simulink model "NoC_4x4x3"  (R2015a)
settings: Solver=ode45  StartTime=0.0  StopTime=10.0  RelTol=1e-3
undefined symbols (not defined in the file or in its folder): des, SELECT
undefined symbols (not defined in the file): MAX, MIN, T
libraries: simulink x48
(part 9 of 12)

== system NoC_4x4x3/LayerUp/Sitch3DXYZ8 ==
  FIFO Queue{,1..6} (7 alike) : FIFOQueue
  Output Switch1 : OutputSwitch  NumberOutputPorts=7  SwitchingCriterion=From attribute  AttributeName=RT  InitialConditionsOpt=on  InitialConditions=5
  Path Combiner : PathCombiner  NumberInputPorts=7  InputPortPrecedence=Equiprobable  InitialSeed=13103
  RouteXYZ : Subsystem
  Single Server1 : SingleServer  ServiceTime=D  StatNumberDeparted=on
  Out_N : PMIOPort  Port=1  Side=Right
  In_N : PMIOPort  Port=2  Side=Left
  In_S : PMIOPort  Port=3  Side=Left
  Out_S : PMIOPort  Port=4  Side=Right
  In_W : PMIOPort  Port=5  Side=Left
  Out_W : PMIOPort  Port=6  Side=Right
  In_E : PMIOPort  Port=7  Side=Left
  Out_E : PMIOPort  Port=8  Side=Right
  In_U : PMIOPort  Port=9  Side=Left
  Out_U : PMIOPort  Port=10  Side=Right
  In_D : PMIOPort  Port=11  Side=Left
  In_NI : PMIOPort  Port=12  Side=Left
  Out_D : PMIOPort  Port=13  Side=Right
  Out_NI : PMIOPort  Port=14  Side=Right
  connections:
  Single Server1/LConn1 -- RouteXYZ/RConn1
  Path Combiner/RConn1 -- RouteXYZ/LConn1
  FIFO Queue6/LConn1 -- In_NI/RConn1
  FIFO Queue5/LConn1 -- In_D/RConn1
  Output Switch1/RConn7 -- Out_NI/RConn1
  Output Switch1/RConn6 -- Out_D/RConn1
  Path Combiner/LConn7 -- FIFO Queue6/RConn1
  Path Combiner/LConn6 -- FIFO Queue5/RConn1
  Out_U/RConn1 -- Output Switch1/RConn5
  Out_E/RConn1 -- Output Switch1/RConn4
  Out_W/RConn1 -- Output Switch1/RConn3
  Out_S/RConn1 -- Output Switch1/RConn2
  Out_N/RConn1 -- Output Switch1/RConn1
  Path Combiner/LConn5 -- FIFO Queue4/RConn1
  Path Combiner/LConn4 -- FIFO Queue3/RConn1
  Path Combiner/LConn3 -- FIFO Queue2/RConn1
  Path Combiner/LConn2 -- FIFO Queue1/RConn1
  Path Combiner/LConn1 -- FIFO Queue/RConn1
  Output Switch1/LConn1 -- Single Server1/RConn1
  FIFO Queue4/LConn1 -- In_U/RConn1
  FIFO Queue/LConn1 -- In_N/RConn1
  FIFO Queue3/LConn1 -- In_E/RConn1
  FIFO Queue2/LConn1 -- In_W/RConn1
  FIFO Queue1/LConn1 -- In_S/RConn1

== system NoC_4x4x3/LayerUp/Sitch3DXYZ9 ==
  FIFO Queue{,1..6} (7 alike) : FIFOQueue
  Output Switch1 : OutputSwitch  NumberOutputPorts=7  SwitchingCriterion=From attribute  AttributeName=RT  InitialConditionsOpt=on  InitialConditions=5
  Path Combiner : PathCombiner  NumberInputPorts=7  InputPortPrecedence=Equiprobable  InitialSeed=6669
  RouteXYZ : Subsystem
  Single Server1 : SingleServer  ServiceTime=D  StatNumberDeparted=on
  Out_N : PMIOPort  Port=1  Side=Right
  In_N : PMIOPort  Port=2  Side=Left
  In_S : PMIOPort  Port=3  Side=Left
  Out_S : PMIOPort  Port=4  Side=Right
  In_W : PMIOPort  Port=5  Side=Left
  Out_W : PMIOPort  Port=6  Side=Right
  In_E : PMIOPort  Port=7  Side=Left
  Out_E : PMIOPort  Port=8  Side=Right
  In_U : PMIOPort  Port=9  Side=Left
  Out_U : PMIOPort  Port=10  Side=Right
  In_D : PMIOPort  Port=11  Side=Left
  In_NI : PMIOPort  Port=12  Side=Left
  Out_D : PMIOPort  Port=13  Side=Right
  Out_NI : PMIOPort  Port=14  Side=Right
  connections:
  FIFO Queue1/LConn1 -- In_S/RConn1
  FIFO Queue2/LConn1 -- In_W/RConn1
  FIFO Queue3/LConn1 -- In_E/RConn1
  FIFO Queue/LConn1 -- In_N/RConn1
  FIFO Queue4/LConn1 -- In_U/RConn1
  Output Switch1/LConn1 -- Single Server1/RConn1
  Path Combiner/LConn1 -- FIFO Queue/RConn1
  Path Combiner/LConn2 -- FIFO Queue1/RConn1
  Path Combiner/LConn3 -- FIFO Queue2/RConn1
  Path Combiner/LConn4 -- FIFO Queue3/RConn1
  Path Combiner/LConn5 -- FIFO Queue4/RConn1
  Out_N/RConn1 -- Output Switch1/RConn1
  Out_S/RConn1 -- Output Switch1/RConn2
  Out_W/RConn1 -- Output Switch1/RConn3
  Out_E/RConn1 -- Output Switch1/RConn4
  Out_U/RConn1 -- Output Switch1/RConn5
  Path Combiner/LConn6 -- FIFO Queue5/RConn1
  Path Combiner/LConn7 -- FIFO Queue6/RConn1
  Output Switch1/RConn6 -- Out_D/RConn1
  Output Switch1/RConn7 -- Out_NI/RConn1
  FIFO Queue5/LConn1 -- In_D/RConn1
  FIFO Queue6/LConn1 -- In_NI/RConn1
  Path Combiner/RConn1 -- RouteXYZ/LConn1
  Single Server1/LConn1 -- RouteXYZ/RConn1

== system NoC_4x4x3/Layer/PE00/Create Generator Selection Variable ==
  function : TriggerPort  TriggerType=function-call
  Repeating Sequence Stair : simulink/Sources/Repeating Sequence Stair  OutValues=[0 1].'  tsamp=-1  OutMin=[]  OutMax=[]  OutDataTypeStr=float('double')  OutputDataTypeScalingMode=Specify via dialog  OutDataType=float('double')  ConRadixGroup=Best Precision: Vector-wise  OutScaling=2^-12
  Out1 : Outport
  wires:
  Repeating Sequence Stair/1 -> Out1/1

== system NoC_4x4x3/Layer/PE01/Create Generator Selection Variable ==
  function : TriggerPort  TriggerType=function-call
  Repeating Sequence Stair : simulink/Sources/Repeating Sequence Stair  OutValues=[0 1].'  tsamp=-1  OutMin=[]  OutMax=[]  OutDataTypeStr=float('double')  OutputDataTypeScalingMode=Specify via dialog  OutDataType=float('double')  ConRadixGroup=Best Precision: Vector-wise  OutScaling=2^-12
  Out1 : Outport
  wires:
  Repeating Sequence Stair/1 -> Out1/1

== system NoC_4x4x3/Layer/PE02/Create Generator Selection Variable ==
  function : TriggerPort  TriggerType=function-call
  Repeating Sequence Stair : simulink/Sources/Repeating Sequence Stair  OutValues=[0 1].'  tsamp=-1  OutMin=[]  OutMax=[]  OutDataTypeStr=float('double')  OutputDataTypeScalingMode=Specify via dialog  OutDataType=float('double')  ConRadixGroup=Best Precision: Vector-wise  OutScaling=2^-12
  Out1 : Outport
  wires:
  Repeating Sequence Stair/1 -> Out1/1

== system NoC_4x4x3/Layer/PE03/Create Generator Selection Variable ==
  function : TriggerPort  TriggerType=function-call
  Repeating Sequence Stair : simulink/Sources/Repeating Sequence Stair  OutValues=[0 1].'  tsamp=-1  OutMin=[]  OutMax=[]  OutDataTypeStr=float('double')  OutputDataTypeScalingMode=Specify via dialog  OutDataType=float('double')  ConRadixGroup=Best Precision: Vector-wise  OutScaling=2^-12
  Out1 : Outport
  wires:
  Repeating Sequence Stair/1 -> Out1/1

== system NoC_4x4x3/Layer/PE10/Create Generator Selection Variable ==
  function : TriggerPort  TriggerType=function-call
  Repeating Sequence Stair : simulink/Sources/Repeating Sequence Stair  OutValues=[0 1].'  tsamp=-1  OutMin=[]  OutMax=[]  OutDataTypeStr=float('double')  OutputDataTypeScalingMode=Specify via dialog  OutDataType=float('double')  ConRadixGroup=Best Precision: Vector-wise  OutScaling=2^-12
  Out1 : Outport
  wires:
  Repeating Sequence Stair/1 -> Out1/1

== system NoC_4x4x3/Layer/PE11/Create Generator Selection Variable ==
  function : TriggerPort  TriggerType=function-call
  Repeating Sequence Stair : simulink/Sources/Repeating Sequence Stair  OutValues=[0 1].'  tsamp=-1  OutMin=[]  OutMax=[]  OutDataTypeStr=float('double')  OutputDataTypeScalingMode=Specify via dialog  OutDataType=float('double')  ConRadixGroup=Best Precision: Vector-wise  OutScaling=2^-12
  Out1 : Outport
  wires:
  Repeating Sequence Stair/1 -> Out1/1

== system NoC_4x4x3/Layer/PE12/Create Generator Selection Variable ==
  function : TriggerPort  TriggerType=function-call
  Repeating Sequence Stair : simulink/Sources/Repeating Sequence Stair  OutValues=[0 1].'  tsamp=-1  OutMin=[]  OutMax=[]  OutDataTypeStr=float('double')  OutputDataTypeScalingMode=Specify via dialog  OutDataType=float('double')  ConRadixGroup=Best Precision: Vector-wise  OutScaling=2^-12
  Out1 : Outport
  wires:
  Repeating Sequence Stair/1 -> Out1/1

== system NoC_4x4x3/Layer/PE13/Create Generator Selection Variable ==
  function : TriggerPort  TriggerType=function-call
  Repeating Sequence Stair : simulink/Sources/Repeating Sequence Stair  OutValues=[0 1].'  tsamp=-1  OutMin=[]  OutMax=[]  OutDataTypeStr=float('double')  OutputDataTypeScalingMode=Specify via dialog  OutDataType=float('double')  ConRadixGroup=Best Precision: Vector-wise  OutScaling=2^-12
  Out1 : Outport
  wires:
  Repeating Sequence Stair/1 -> Out1/1

== system NoC_4x4x3/Layer/PE20/Create Generator Selection Variable ==
  function : TriggerPort  TriggerType=function-call
  Repeating Sequence Stair : simulink/Sources/Repeating Sequence Stair  OutValues=[0 1].'  tsamp=-1  OutMin=[]  OutMax=[]  OutDataTypeStr=float('double')  OutputDataTypeScalingMode=Specify via dialog  OutDataType=float('double')  ConRadixGroup=Best Precision: Vector-wise  OutScaling=2^-12
  Out1 : Outport
  wires:
  Repeating Sequence Stair/1 -> Out1/1

== system NoC_4x4x3/Layer/PE21/Create Generator Selection Variable ==
  function : TriggerPort  TriggerType=function-call
  Repeating Sequence Stair : simulink/Sources/Repeating Sequence Stair  OutValues=[0 1].'  tsamp=-1  OutMin=[]  OutMax=[]  OutDataTypeStr=float('double')  OutputDataTypeScalingMode=Specify via dialog  OutDataType=float('double')  ConRadixGroup=Best Precision: Vector-wise  OutScaling=2^-12
  Out1 : Outport
  wires:
  Repeating Sequence Stair/1 -> Out1/1

== system NoC_4x4x3/Layer/PE22/Create Generator Selection Variable ==
  function : TriggerPort  TriggerType=function-call
  Repeating Sequence Stair : simulink/Sources/Repeating Sequence Stair  OutValues=[0 1].'  tsamp=-1  OutMin=[]  OutMax=[]  OutDataTypeStr=float('double')  OutputDataTypeScalingMode=Specify via dialog  OutDataType=float('double')  ConRadixGroup=Best Precision: Vector-wise  OutScaling=2^-12
  Out1 : Outport
  wires:
  Repeating Sequence Stair/1 -> Out1/1

== system NoC_4x4x3/Layer/PE23/Create Generator Selection Variable ==
  function : TriggerPort  TriggerType=function-call
  Repeating Sequence Stair : simulink/Sources/Repeating Sequence Stair  OutValues=[0 1].'  tsamp=-1  OutMin=[]  OutMax=[]  OutDataTypeStr=float('double')  OutputDataTypeScalingMode=Specify via dialog  OutDataType=float('double')  ConRadixGroup=Best Precision: Vector-wise  OutScaling=2^-12
  Out1 : Outport
  wires:
  Repeating Sequence Stair/1 -> Out1/1

== system NoC_4x4x3/Layer/PE30/Create Generator Selection Variable ==
  function : TriggerPort  TriggerType=function-call
  Repeating Sequence Stair : simulink/Sources/Repeating Sequence Stair  OutValues=[0 1].'  tsamp=-1  OutMin=[]  OutMax=[]  OutDataTypeStr=float('double')  OutputDataTypeScalingMode=Specify via dialog  OutDataType=float('double')  ConRadixGroup=Best Precision: Vector-wise  OutScaling=2^-12
  Out1 : Outport
  wires:
  Repeating Sequence Stair/1 -> Out1/1

== system NoC_4x4x3/Layer/PE31/Create Generator Selection Variable ==
  function : TriggerPort  TriggerType=function-call
  Repeating Sequence Stair : simulink/Sources/Repeating Sequence Stair  OutValues=[0 1].'  tsamp=-1  OutMin=[]  OutMax=[]  OutDataTypeStr=float('double')  OutputDataTypeScalingMode=Specify via dialog  OutDataType=float('double')  ConRadixGroup=Best Precision: Vector-wise  OutScaling=2^-12
  Out1 : Outport
  wires:
  Repeating Sequence Stair/1 -> Out1/1

== system NoC_4x4x3/Layer/PE32/Create Generator Selection Variable ==
  function : TriggerPort  TriggerType=function-call
  Repeating Sequence Stair : simulink/Sources/Repeating Sequence Stair  OutValues=[0 1].'  tsamp=-1  OutMin=[]  OutMax=[]  OutDataTypeStr=float('double')  OutputDataTypeScalingMode=Specify via dialog  OutDataType=float('double')  ConRadixGroup=Best Precision: Vector-wise  OutScaling=2^-12
  Out1 : Outport
  wires:
  Repeating Sequence Stair/1 -> Out1/1

== system NoC_4x4x3/Layer/PE33/Create Generator Selection Variable ==
  function : TriggerPort  TriggerType=function-call
  Repeating Sequence Stair : simulink/Sources/Repeating Sequence Stair  OutValues=[0 1].'  tsamp=-1  OutMin=[]  OutMax=[]  OutDataTypeStr=float('double')  OutputDataTypeScalingMode=Specify via dialog  OutDataType=float('double')  ConRadixGroup=Best Precision: Vector-wise  OutScaling=2^-12
  Out1 : Outport
  wires:
  Repeating Sequence Stair/1 -> Out1/1

== system NoC_4x4x3/Layer/Sitch3DXYZ/RouteXYZ ==
  Attribute Function : Subsystem  LoadFcn=des.afb.attributefunction_support(gcb,'LoadFcn');  StartFcn=des.afb.attributefunction_support(gcb,'StartFcn');  mask(Attribute Function){OutputNamePrefix=out_}
      mask prompts: OutputNamePrefix "Prefix name"
      settings: CopyFcn=des.afb.attributefunction_support(gcb,'CopyFcn');  OpenFcn=des.afb.attributefunction_support(gcb,'OpenFcn');  ErrorFcn=des.afb.error_redirect
      mask Help: slhelp(gcbh)
      mask Display: image(des_iconLoad('attribFunction.jpg'),'center');
  Set Attribute : SetAttribute  AttributeName=IME_X|IME_Y|IME_Z  AttributeFrom=Dialog|Dialog|Dialog  AttributeValue=ME_X|ME_Y|ME_Z  AttributeTreatAsVector=1|1|1  EvaluatedAttributeValue={ ME_X;ME_Y;ME_Z}
  Input : PMIOPort  Port=1  Side=Left
  Output : PMIOPort  Port=2  Side=Right
  connections:
  Set Attribute/RConn1 -- Attribute Function/LConn1
  Output/RConn1 -- Attribute Function/RConn1
  Input/RConn1 -- Set Attribute/LConn1

== system NoC_4x4x3/Layer/Sitch3DXYZ1/RouteXYZ ==
  Attribute Function : Subsystem  LoadFcn=des.afb.attributefunction_support(gcb,'LoadFcn');  StartFcn=des.afb.attributefunction_support(gcb,'StartFcn');  mask(Attribute Function){OutputNamePrefix=out_}
      mask prompts: OutputNamePrefix "Prefix name"
      settings: CopyFcn=des.afb.attributefunction_support(gcb,'CopyFcn');  OpenFcn=des.afb.attributefunction_support(gcb,'OpenFcn');  ErrorFcn=des.afb.error_redirect
      mask Help: slhelp(gcbh)
      mask Display: image(des_iconLoad('attribFunction.jpg'),'center');
  Set Attribute : SetAttribute  AttributeName=IME_X|IME_Y|IME_Z  AttributeFrom=Dialog|Dialog|Dialog  AttributeValue=ME_X|ME_Y|ME_Z  AttributeTreatAsVector=1|1|1  EvaluatedAttributeValue={ ME_X;ME_Y;ME_Z}
  Input : PMIOPort  Port=1  Side=Left
  Output : PMIOPort  Port=2  Side=Right
  connections:
  Input/RConn1 -- Set Attribute/LConn1
  Output/RConn1 -- Attribute Function/RConn1
  Set Attribute/RConn1 -- Attribute Function/LConn1

== system NoC_4x4x3/Layer/Sitch3DXYZ10/RouteXYZ ==
  Attribute Function : Subsystem  LoadFcn=des.afb.attributefunction_support(gcb,'LoadFcn');  StartFcn=des.afb.attributefunction_support(gcb,'StartFcn');  mask(Attribute Function){OutputNamePrefix=out_}
      mask prompts: OutputNamePrefix "Prefix name"
      settings: CopyFcn=des.afb.attributefunction_support(gcb,'CopyFcn');  OpenFcn=des.afb.attributefunction_support(gcb,'OpenFcn');  ErrorFcn=des.afb.error_redirect
      mask Help: slhelp(gcbh)
      mask Display: image(des_iconLoad('attribFunction.jpg'),'center');
  Set Attribute : SetAttribute  AttributeName=IME_X|IME_Y|IME_Z  AttributeFrom=Dialog|Dialog|Dialog  AttributeValue=ME_X|ME_Y|ME_Z  AttributeTreatAsVector=1|1|1  EvaluatedAttributeValue={ ME_X;ME_Y;ME_Z}
  Input : PMIOPort  Port=1  Side=Left
  Output : PMIOPort  Port=2  Side=Right
  connections:
  Set Attribute/RConn1 -- Attribute Function/LConn1
  Output/RConn1 -- Attribute Function/RConn1
  Input/RConn1 -- Set Attribute/LConn1

== system NoC_4x4x3/Layer/Sitch3DXYZ11/RouteXYZ ==
  Attribute Function : Subsystem  LoadFcn=des.afb.attributefunction_support(gcb,'LoadFcn');  StartFcn=des.afb.attributefunction_support(gcb,'StartFcn');  mask(Attribute Function){OutputNamePrefix=out_}
      mask prompts: OutputNamePrefix "Prefix name"
      settings: CopyFcn=des.afb.attributefunction_support(gcb,'CopyFcn');  OpenFcn=des.afb.attributefunction_support(gcb,'OpenFcn');  ErrorFcn=des.afb.error_redirect
      mask Help: slhelp(gcbh)
      mask Display: image(des_iconLoad('attribFunction.jpg'),'center');
  Set Attribute : SetAttribute  AttributeName=IME_X|IME_Y|IME_Z  AttributeFrom=Dialog|Dialog|Dialog  AttributeValue=ME_X|ME_Y|ME_Z  AttributeTreatAsVector=1|1|1  EvaluatedAttributeValue={ ME_X;ME_Y;ME_Z}
  Input : PMIOPort  Port=1  Side=Left
  Output : PMIOPort  Port=2  Side=Right
  connections:
  Input/RConn1 -- Set Attribute/LConn1
  Output/RConn1 -- Attribute Function/RConn1
  Set Attribute/RConn1 -- Attribute Function/LConn1

== system NoC_4x4x3/Layer/Sitch3DXYZ12/RouteXYZ ==
  Attribute Function : Subsystem  LoadFcn=des.afb.attributefunction_support(gcb,'LoadFcn');  StartFcn=des.afb.attributefunction_support(gcb,'StartFcn');  mask(Attribute Function){OutputNamePrefix=out_}
      mask prompts: OutputNamePrefix "Prefix name"
      settings: CopyFcn=des.afb.attributefunction_support(gcb,'CopyFcn');  OpenFcn=des.afb.attributefunction_support(gcb,'OpenFcn');  ErrorFcn=des.afb.error_redirect
      mask Help: slhelp(gcbh)
      mask Display: image(des_iconLoad('attribFunction.jpg'),'center');
  Set Attribute : SetAttribute  AttributeName=IME_X|IME_Y|IME_Z  AttributeFrom=Dialog|Dialog|Dialog  AttributeValue=ME_X|ME_Y|ME_Z  AttributeTreatAsVector=1|1|1  EvaluatedAttributeValue={ ME_X;ME_Y;ME_Z}
  Input : PMIOPort  Port=1  Side=Left
  Output : PMIOPort  Port=2  Side=Right
  connections:
  Input/RConn1 -- Set Attribute/LConn1
  Output/RConn1 -- Attribute Function/RConn1
  Set Attribute/RConn1 -- Attribute Function/LConn1

== system NoC_4x4x3/Layer/Sitch3DXYZ13/RouteXYZ ==
  Attribute Function : Subsystem  LoadFcn=des.afb.attributefunction_support(gcb,'LoadFcn');  StartFcn=des.afb.attributefunction_support(gcb,'StartFcn');  mask(Attribute Function){OutputNamePrefix=out_}
      mask prompts: OutputNamePrefix "Prefix name"
      settings: CopyFcn=des.afb.attributefunction_support(gcb,'CopyFcn');  OpenFcn=des.afb.attributefunction_support(gcb,'OpenFcn');  ErrorFcn=des.afb.error_redirect
      mask Help: slhelp(gcbh)
      mask Display: image(des_iconLoad('attribFunction.jpg'),'center');
  Set Attribute : SetAttribute  AttributeName=IME_X|IME_Y|IME_Z  AttributeFrom=Dialog|Dialog|Dialog  AttributeValue=ME_X|ME_Y|ME_Z  AttributeTreatAsVector=1|1|1  EvaluatedAttributeValue={ ME_X;ME_Y;ME_Z}
  Input : PMIOPort  Port=1  Side=Left
  Output : PMIOPort  Port=2  Side=Right
  connections:
  Set Attribute/RConn1 -- Attribute Function/LConn1
  Output/RConn1 -- Attribute Function/RConn1
  Input/RConn1 -- Set Attribute/LConn1

== system NoC_4x4x3/Layer/Sitch3DXYZ14/RouteXYZ ==
  Attribute Function : Subsystem  LoadFcn=des.afb.attributefunction_support(gcb,'LoadFcn');  StartFcn=des.afb.attributefunction_support(gcb,'StartFcn');  mask(Attribute Function){OutputNamePrefix=out_}
      mask prompts: OutputNamePrefix "Prefix name"
      settings: CopyFcn=des.afb.attributefunction_support(gcb,'CopyFcn');  OpenFcn=des.afb.attributefunction_support(gcb,'OpenFcn');  ErrorFcn=des.afb.error_redirect
      mask Help: slhelp(gcbh)
      mask Display: image(des_iconLoad('attribFunction.jpg'),'center');
  Set Attribute : SetAttribute  AttributeName=IME_X|IME_Y|IME_Z  AttributeFrom=Dialog|Dialog|Dialog  AttributeValue=ME_X|ME_Y|ME_Z  AttributeTreatAsVector=1|1|1  EvaluatedAttributeValue={ ME_X;ME_Y;ME_Z}
  Input : PMIOPort  Port=1  Side=Left
  Output : PMIOPort  Port=2  Side=Right
  connections:
  Input/RConn1 -- Set Attribute/LConn1
  Output/RConn1 -- Attribute Function/RConn1
  Set Attribute/RConn1 -- Attribute Function/LConn1

== system NoC_4x4x3/Layer/Sitch3DXYZ15/RouteXYZ ==
  Attribute Function : Subsystem  LoadFcn=des.afb.attributefunction_support(gcb,'LoadFcn');  StartFcn=des.afb.attributefunction_support(gcb,'StartFcn');  mask(Attribute Function){OutputNamePrefix=out_}
      mask prompts: OutputNamePrefix "Prefix name"
      settings: CopyFcn=des.afb.attributefunction_support(gcb,'CopyFcn');  OpenFcn=des.afb.attributefunction_support(gcb,'OpenFcn');  ErrorFcn=des.afb.error_redirect
      mask Help: slhelp(gcbh)
      mask Display: image(des_iconLoad('attribFunction.jpg'),'center');
  Set Attribute : SetAttribute  AttributeName=IME_X|IME_Y|IME_Z  AttributeFrom=Dialog|Dialog|Dialog  AttributeValue=ME_X|ME_Y|ME_Z  AttributeTreatAsVector=1|1|1  EvaluatedAttributeValue={ ME_X;ME_Y;ME_Z}
  Input : PMIOPort  Port=1  Side=Left
  Output : PMIOPort  Port=2  Side=Right
  connections:
  Set Attribute/RConn1 -- Attribute Function/LConn1
  Output/RConn1 -- Attribute Function/RConn1
  Input/RConn1 -- Set Attribute/LConn1

== system NoC_4x4x3/Layer/Sitch3DXYZ2/RouteXYZ ==
  Attribute Function : Subsystem  LoadFcn=des.afb.attributefunction_support(gcb,'LoadFcn');  StartFcn=des.afb.attributefunction_support(gcb,'StartFcn');  mask(Attribute Function){OutputNamePrefix=out_}
      mask prompts: OutputNamePrefix "Prefix name"
      settings: CopyFcn=des.afb.attributefunction_support(gcb,'CopyFcn');  OpenFcn=des.afb.attributefunction_support(gcb,'OpenFcn');  ErrorFcn=des.afb.error_redirect
      mask Help: slhelp(gcbh)
      mask Display: image(des_iconLoad('attribFunction.jpg'),'center');
  Set Attribute : SetAttribute  AttributeName=IME_X|IME_Y|IME_Z  AttributeFrom=Dialog|Dialog|Dialog  AttributeValue=ME_X|ME_Y|ME_Z  AttributeTreatAsVector=1|1|1  EvaluatedAttributeValue={ ME_X;ME_Y;ME_Z}
  Input : PMIOPort  Port=1  Side=Left
  Output : PMIOPort  Port=2  Side=Right
  connections:
  Set Attribute/RConn1 -- Attribute Function/LConn1
  Output/RConn1 -- Attribute Function/RConn1
  Input/RConn1 -- Set Attribute/LConn1

== system NoC_4x4x3/Layer/Sitch3DXYZ3/RouteXYZ ==
  Attribute Function : Subsystem  LoadFcn=des.afb.attributefunction_support(gcb,'LoadFcn');  StartFcn=des.afb.attributefunction_support(gcb,'StartFcn');  mask(Attribute Function){OutputNamePrefix=out_}
      mask prompts: OutputNamePrefix "Prefix name"
      settings: CopyFcn=des.afb.attributefunction_support(gcb,'CopyFcn');  OpenFcn=des.afb.attributefunction_support(gcb,'OpenFcn');  ErrorFcn=des.afb.error_redirect
      mask Help: slhelp(gcbh)
      mask Display: image(des_iconLoad('attribFunction.jpg'),'center');
  Set Attribute : SetAttribute  AttributeName=IME_X|IME_Y|IME_Z  AttributeFrom=Dialog|Dialog|Dialog  AttributeValue=ME_X|ME_Y|ME_Z  AttributeTreatAsVector=1|1|1  EvaluatedAttributeValue={ ME_X;ME_Y;ME_Z}
  Input : PMIOPort  Port=1  Side=Left
  Output : PMIOPort  Port=2  Side=Right
  connections:
  Input/RConn1 -- Set Attribute/LConn1
  Output/RConn1 -- Attribute Function/RConn1
  Set Attribute/RConn1 -- Attribute Function/LConn1

== system NoC_4x4x3/Layer/Sitch3DXYZ4/RouteXYZ ==
  Attribute Function : Subsystem  LoadFcn=des.afb.attributefunction_support(gcb,'LoadFcn');  StartFcn=des.afb.attributefunction_support(gcb,'StartFcn');  mask(Attribute Function){OutputNamePrefix=out_}
      mask prompts: OutputNamePrefix "Prefix name"
      settings: CopyFcn=des.afb.attributefunction_support(gcb,'CopyFcn');  OpenFcn=des.afb.attributefunction_support(gcb,'OpenFcn');  ErrorFcn=des.afb.error_redirect
      mask Help: slhelp(gcbh)
      mask Display: image(des_iconLoad('attribFunction.jpg'),'center');
  Set Attribute : SetAttribute  AttributeName=IME_X|IME_Y|IME_Z  AttributeFrom=Dialog|Dialog|Dialog  AttributeValue=ME_X|ME_Y|ME_Z  AttributeTreatAsVector=1|1|1  EvaluatedAttributeValue={ ME_X;ME_Y;ME_Z}
  Input : PMIOPort  Port=1  Side=Left
  Output : PMIOPort  Port=2  Side=Right
  connections:
  Input/RConn1 -- Set Attribute/LConn1
  Output/RConn1 -- Attribute Function/RConn1
  Set Attribute/RConn1 -- Attribute Function/LConn1

== system NoC_4x4x3/Layer/Sitch3DXYZ5/RouteXYZ ==
  Attribute Function : Subsystem  LoadFcn=des.afb.attributefunction_support(gcb,'LoadFcn');  StartFcn=des.afb.attributefunction_support(gcb,'StartFcn');  mask(Attribute Function){OutputNamePrefix=out_}
      mask prompts: OutputNamePrefix "Prefix name"
      settings: CopyFcn=des.afb.attributefunction_support(gcb,'CopyFcn');  OpenFcn=des.afb.attributefunction_support(gcb,'OpenFcn');  ErrorFcn=des.afb.error_redirect
      mask Help: slhelp(gcbh)
      mask Display: image(des_iconLoad('attribFunction.jpg'),'center');
  Set Attribute : SetAttribute  AttributeName=IME_X|IME_Y|IME_Z  AttributeFrom=Dialog|Dialog|Dialog  AttributeValue=ME_X|ME_Y|ME_Z  AttributeTreatAsVector=1|1|1  EvaluatedAttributeValue={ ME_X;ME_Y;ME_Z}
  Input : PMIOPort  Port=1  Side=Left
  Output : PMIOPort  Port=2  Side=Right
  connections:
  Set Attribute/RConn1 -- Attribute Function/LConn1
  Output/RConn1 -- Attribute Function/RConn1
  Input/RConn1 -- Set Attribute/LConn1

== system NoC_4x4x3/Layer/Sitch3DXYZ6/RouteXYZ ==
  Attribute Function : Subsystem  LoadFcn=des.afb.attributefunction_support(gcb,'LoadFcn');  StartFcn=des.afb.attributefunction_support(gcb,'StartFcn');  mask(Attribute Function){OutputNamePrefix=out_}
      mask prompts: OutputNamePrefix "Prefix name"
      settings: CopyFcn=des.afb.attributefunction_support(gcb,'CopyFcn');  OpenFcn=des.afb.attributefunction_support(gcb,'OpenFcn');  ErrorFcn=des.afb.error_redirect
      mask Help: slhelp(gcbh)
      mask Display: image(des_iconLoad('attribFunction.jpg'),'center');
  Set Attribute : SetAttribute  AttributeName=IME_X|IME_Y|IME_Z  AttributeFrom=Dialog|Dialog|Dialog  AttributeValue=ME_X|ME_Y|ME_Z  AttributeTreatAsVector=1|1|1  EvaluatedAttributeValue={ ME_X;ME_Y;ME_Z}
  Input : PMIOPort  Port=1  Side=Left
  Output : PMIOPort  Port=2  Side=Right
  connections:
  Input/RConn1 -- Set Attribute/LConn1
  Output/RConn1 -- Attribute Function/RConn1
  Set Attribute/RConn1 -- Attribute Function/LConn1

== system NoC_4x4x3/Layer/Sitch3DXYZ7/RouteXYZ ==
  Attribute Function : Subsystem  LoadFcn=des.afb.attributefunction_support(gcb,'LoadFcn');  StartFcn=des.afb.attributefunction_support(gcb,'StartFcn');  mask(Attribute Function){OutputNamePrefix=out_}
      mask prompts: OutputNamePrefix "Prefix name"
      settings: CopyFcn=des.afb.attributefunction_support(gcb,'CopyFcn');  OpenFcn=des.afb.attributefunction_support(gcb,'OpenFcn');  ErrorFcn=des.afb.error_redirect
      mask Help: slhelp(gcbh)
      mask Display: image(des_iconLoad('attribFunction.jpg'),'center');
  Set Attribute : SetAttribute  AttributeName=IME_X|IME_Y|IME_Z  AttributeFrom=Dialog|Dialog|Dialog  AttributeValue=ME_X|ME_Y|ME_Z  AttributeTreatAsVector=1|1|1  EvaluatedAttributeValue={ ME_X;ME_Y;ME_Z}
  Input : PMIOPort  Port=1  Side=Left
  Output : PMIOPort  Port=2  Side=Right
  connections:
  Set Attribute/RConn1 -- Attribute Function/LConn1
  Output/RConn1 -- Attribute Function/RConn1
  Input/RConn1 -- Set Attribute/LConn1

== system NoC_4x4x3/Layer/Sitch3DXYZ8/RouteXYZ ==
  Attribute Function : Subsystem  LoadFcn=des.afb.attributefunction_support(gcb,'LoadFcn');  StartFcn=des.afb.attributefunction_support(gcb,'StartFcn');  mask(Attribute Function){OutputNamePrefix=out_}
      mask prompts: OutputNamePrefix "Prefix name"
      settings: CopyFcn=des.afb.attributefunction_support(gcb,'CopyFcn');  OpenFcn=des.afb.attributefunction_support(gcb,'OpenFcn');  ErrorFcn=des.afb.error_redirect
      mask Help: slhelp(gcbh)
      mask Display: image(des_iconLoad('attribFunction.jpg'),'center');
  Set Attribute : SetAttribute  AttributeName=IME_X|IME_Y|IME_Z  AttributeFrom=Dialog|Dialog|Dialog  AttributeValue=ME_X|ME_Y|ME_Z  AttributeTreatAsVector=1|1|1  EvaluatedAttributeValue={ ME_X;ME_Y;ME_Z}
  Input : PMIOPort  Port=1  Side=Left
  Output : PMIOPort  Port=2  Side=Right
  connections:
  Set Attribute/RConn1 -- Attribute Function/LConn1
  Output/RConn1 -- Attribute Function/RConn1
  Input/RConn1 -- Set Attribute/LConn1

== system NoC_4x4x3/Layer/Sitch3DXYZ9/RouteXYZ ==
  Attribute Function : Subsystem  LoadFcn=des.afb.attributefunction_support(gcb,'LoadFcn');  StartFcn=des.afb.attributefunction_support(gcb,'StartFcn');  mask(Attribute Function){OutputNamePrefix=out_}
      mask prompts: OutputNamePrefix "Prefix name"
      settings: CopyFcn=des.afb.attributefunction_support(gcb,'CopyFcn');  OpenFcn=des.afb.attributefunction_support(gcb,'OpenFcn');  ErrorFcn=des.afb.error_redirect
      mask Help: slhelp(gcbh)
      mask Display: image(des_iconLoad('attribFunction.jpg'),'center');
  Set Attribute : SetAttribute  AttributeName=IME_X|IME_Y|IME_Z  AttributeFrom=Dialog|Dialog|Dialog  AttributeValue=ME_X|ME_Y|ME_Z  AttributeTreatAsVector=1|1|1  EvaluatedAttributeValue={ ME_X;ME_Y;ME_Z}
  Input : PMIOPort  Port=1  Side=Left
  Output : PMIOPort  Port=2  Side=Right
  connections:
  Input/RConn1 -- Set Attribute/LConn1
  Output/RConn1 -- Attribute Function/RConn1
  Set Attribute/RConn1 -- Attribute Function/LConn1

== system NoC_4x4x3/LayerDown/PE00/Create Generator Selection Variable ==
  function : TriggerPort  TriggerType=function-call
  Repeating Sequence Stair : simulink/Sources/Repeating Sequence Stair  OutValues=[0 1].'  tsamp=-1  OutMin=[]  OutMax=[]  OutDataTypeStr=float('double')  OutputDataTypeScalingMode=Specify via dialog  OutDataType=float('double')  ConRadixGroup=Best Precision: Vector-wise  OutScaling=2^-12
  Out1 : Outport
  wires:
  Repeating Sequence Stair/1 -> Out1/1

== system NoC_4x4x3/LayerDown/PE01/Create Generator Selection Variable ==
  function : TriggerPort  TriggerType=function-call
  Repeating Sequence Stair : simulink/Sources/Repeating Sequence Stair  OutValues=[0 1].'  tsamp=-1  OutMin=[]  OutMax=[]  OutDataTypeStr=float('double')  OutputDataTypeScalingMode=Specify via dialog  OutDataType=float('double')  ConRadixGroup=Best Precision: Vector-wise  OutScaling=2^-12
  Out1 : Outport
  wires:
  Repeating Sequence Stair/1 -> Out1/1

== system NoC_4x4x3/LayerDown/PE02/Create Generator Selection Variable ==
  function : TriggerPort  TriggerType=function-call
  Repeating Sequence Stair : simulink/Sources/Repeating Sequence Stair  OutValues=[0 1].'  tsamp=-1  OutMin=[]  OutMax=[]  OutDataTypeStr=float('double')  OutputDataTypeScalingMode=Specify via dialog  OutDataType=float('double')  ConRadixGroup=Best Precision: Vector-wise  OutScaling=2^-12
  Out1 : Outport
  wires:
  Repeating Sequence Stair/1 -> Out1/1

== system NoC_4x4x3/LayerDown/PE03/Create Generator Selection Variable ==
  function : TriggerPort  TriggerType=function-call
  Repeating Sequence Stair : simulink/Sources/Repeating Sequence Stair  OutValues=[0 1].'  tsamp=-1  OutMin=[]  OutMax=[]  OutDataTypeStr=float('double')  OutputDataTypeScalingMode=Specify via dialog  OutDataType=float('double')  ConRadixGroup=Best Precision: Vector-wise  OutScaling=2^-12
  Out1 : Outport
  wires:
  Repeating Sequence Stair/1 -> Out1/1

== system NoC_4x4x3/LayerDown/PE10/Create Generator Selection Variable ==
  function : TriggerPort  TriggerType=function-call
  Repeating Sequence Stair : simulink/Sources/Repeating Sequence Stair  OutValues=[0 1].'  tsamp=-1  OutMin=[]  OutMax=[]  OutDataTypeStr=float('double')  OutputDataTypeScalingMode=Specify via dialog  OutDataType=float('double')  ConRadixGroup=Best Precision: Vector-wise  OutScaling=2^-12
  Out1 : Outport
  wires:
  Repeating Sequence Stair/1 -> Out1/1

== system NoC_4x4x3/LayerDown/PE11/Create Generator Selection Variable ==
  function : TriggerPort  TriggerType=function-call
  Repeating Sequence Stair : simulink/Sources/Repeating Sequence Stair  OutValues=[0 1].'  tsamp=-1  OutMin=[]  OutMax=[]  OutDataTypeStr=float('double')  OutputDataTypeScalingMode=Specify via dialog  OutDataType=float('double')  ConRadixGroup=Best Precision: Vector-wise  OutScaling=2^-12
  Out1 : Outport
  wires:
  Repeating Sequence Stair/1 -> Out1/1

== system NoC_4x4x3/LayerDown/PE12/Create Generator Selection Variable ==
  function : TriggerPort  TriggerType=function-call
  Repeating Sequence Stair : simulink/Sources/Repeating Sequence Stair  OutValues=[0 1].'  tsamp=-1  OutMin=[]  OutMax=[]  OutDataTypeStr=float('double')  OutputDataTypeScalingMode=Specify via dialog  OutDataType=float('double')  ConRadixGroup=Best Precision: Vector-wise  OutScaling=2^-12
  Out1 : Outport
  wires:
  Repeating Sequence Stair/1 -> Out1/1

== system NoC_4x4x3/LayerDown/PE13/Create Generator Selection Variable ==
  function : TriggerPort  TriggerType=function-call
  Repeating Sequence Stair : simulink/Sources/Repeating Sequence Stair  OutValues=[0 1].'  tsamp=-1  OutMin=[]  OutMax=[]  OutDataTypeStr=float('double')  OutputDataTypeScalingMode=Specify via dialog  OutDataType=float('double')  ConRadixGroup=Best Precision: Vector-wise  OutScaling=2^-12
  Out1 : Outport
  wires:
  Repeating Sequence Stair/1 -> Out1/1

== system NoC_4x4x3/LayerDown/PE20/Create Generator Selection Variable ==
  function : TriggerPort  TriggerType=function-call
  Repeating Sequence Stair : simulink/Sources/Repeating Sequence Stair  OutValues=[0 1].'  tsamp=-1  OutMin=[]  OutMax=[]  OutDataTypeStr=float('double')  OutputDataTypeScalingMode=Specify via dialog  OutDataType=float('double')  ConRadixGroup=Best Precision: Vector-wise  OutScaling=2^-12
  Out1 : Outport
  wires:
  Repeating Sequence Stair/1 -> Out1/1

== system NoC_4x4x3/LayerDown/PE21/Create Generator Selection Variable ==
  function : TriggerPort  TriggerType=function-call
  Repeating Sequence Stair : simulink/Sources/Repeating Sequence Stair  OutValues=[0 1].'  tsamp=-1  OutMin=[]  OutMax=[]  OutDataTypeStr=float('double')  OutputDataTypeScalingMode=Specify via dialog  OutDataType=float('double')  ConRadixGroup=Best Precision: Vector-wise  OutScaling=2^-12
  Out1 : Outport
  wires:
  Repeating Sequence Stair/1 -> Out1/1

== system NoC_4x4x3/LayerDown/PE22/Create Generator Selection Variable ==
  function : TriggerPort  TriggerType=function-call
  Repeating Sequence Stair : simulink/Sources/Repeating Sequence Stair  OutValues=[0 1].'  tsamp=-1  OutMin=[]  OutMax=[]  OutDataTypeStr=float('double')  OutputDataTypeScalingMode=Specify via dialog  OutDataType=float('double')  ConRadixGroup=Best Precision: Vector-wise  OutScaling=2^-12
  Out1 : Outport
  wires:
  Repeating Sequence Stair/1 -> Out1/1

== system NoC_4x4x3/LayerDown/PE23/Create Generator Selection Variable ==
  function : TriggerPort  TriggerType=function-call
  Repeating Sequence Stair : simulink/Sources/Repeating Sequence Stair  OutValues=[0 1].'  tsamp=-1  OutMin=[]  OutMax=[]  OutDataTypeStr=float('double')  OutputDataTypeScalingMode=Specify via dialog  OutDataType=float('double')  ConRadixGroup=Best Precision: Vector-wise  OutScaling=2^-12
  Out1 : Outport
  wires:
  Repeating Sequence Stair/1 -> Out1/1

== system NoC_4x4x3/LayerDown/PE30/Create Generator Selection Variable ==
  function : TriggerPort  TriggerType=function-call
  Repeating Sequence Stair : simulink/Sources/Repeating Sequence Stair  OutValues=[0 1].'  tsamp=-1  OutMin=[]  OutMax=[]  OutDataTypeStr=float('double')  OutputDataTypeScalingMode=Specify via dialog  OutDataType=float('double')  ConRadixGroup=Best Precision: Vector-wise  OutScaling=2^-12
  Out1 : Outport
  wires:
  Repeating Sequence Stair/1 -> Out1/1

== system NoC_4x4x3/LayerDown/PE31/Create Generator Selection Variable ==
  function : TriggerPort  TriggerType=function-call
  Repeating Sequence Stair : simulink/Sources/Repeating Sequence Stair  OutValues=[0 1].'  tsamp=-1  OutMin=[]  OutMax=[]  OutDataTypeStr=float('double')  OutputDataTypeScalingMode=Specify via dialog  OutDataType=float('double')  ConRadixGroup=Best Precision: Vector-wise  OutScaling=2^-12
  Out1 : Outport
  wires:
  Repeating Sequence Stair/1 -> Out1/1

== system NoC_4x4x3/LayerDown/PE32/Create Generator Selection Variable ==
  function : TriggerPort  TriggerType=function-call
  Repeating Sequence Stair : simulink/Sources/Repeating Sequence Stair  OutValues=[0 1].'  tsamp=-1  OutMin=[]  OutMax=[]  OutDataTypeStr=float('double')  OutputDataTypeScalingMode=Specify via dialog  OutDataType=float('double')  ConRadixGroup=Best Precision: Vector-wise  OutScaling=2^-12
  Out1 : Outport
  wires:
  Repeating Sequence Stair/1 -> Out1/1

== system NoC_4x4x3/LayerDown/PE33/Create Generator Selection Variable ==
  function : TriggerPort  TriggerType=function-call
  Repeating Sequence Stair : simulink/Sources/Repeating Sequence Stair  OutValues=[0 1].'  tsamp=-1  OutMin=[]  OutMax=[]  OutDataTypeStr=float('double')  OutputDataTypeScalingMode=Specify via dialog  OutDataType=float('double')  ConRadixGroup=Best Precision: Vector-wise  OutScaling=2^-12
  Out1 : Outport
  wires:
  Repeating Sequence Stair/1 -> Out1/1

== system NoC_4x4x3/LayerDown/Sitch3DXYZ/RouteXYZ ==
  Attribute Function : Subsystem  LoadFcn=des.afb.attributefunction_support(gcb,'LoadFcn');  StartFcn=des.afb.attributefunction_support(gcb,'StartFcn');  mask(Attribute Function){OutputNamePrefix=out_}
      mask prompts: OutputNamePrefix "Prefix name"
      settings: CopyFcn=des.afb.attributefunction_support(gcb,'CopyFcn');  OpenFcn=des.afb.attributefunction_support(gcb,'OpenFcn');  ErrorFcn=des.afb.error_redirect
      mask Help: slhelp(gcbh)
      mask Display: image(des_iconLoad('attribFunction.jpg'),'center');
  Set Attribute : SetAttribute  AttributeName=IME_X|IME_Y|IME_Z  AttributeFrom=Dialog|Dialog|Dialog  AttributeValue=ME_X|ME_Y|ME_Z  AttributeTreatAsVector=1|1|1  EvaluatedAttributeValue={ ME_X;ME_Y;ME_Z}
  Input : PMIOPort  Port=1  Side=Left
  Output : PMIOPort  Port=2  Side=Right
  connections:
  Input/RConn1 -- Set Attribute/LConn1
  Output/RConn1 -- Attribute Function/RConn1
  Set Attribute/RConn1 -- Attribute Function/LConn1

== system NoC_4x4x3/LayerDown/Sitch3DXYZ1/RouteXYZ ==
  Attribute Function : Subsystem  LoadFcn=des.afb.attributefunction_support(gcb,'LoadFcn');  StartFcn=des.afb.attributefunction_support(gcb,'StartFcn');  mask(Attribute Function){OutputNamePrefix=out_}
      mask prompts: OutputNamePrefix "Prefix name"
      settings: CopyFcn=des.afb.attributefunction_support(gcb,'CopyFcn');  OpenFcn=des.afb.attributefunction_support(gcb,'OpenFcn');  ErrorFcn=des.afb.error_redirect
      mask Help: slhelp(gcbh)
      mask Display: image(des_iconLoad('attribFunction.jpg'),'center');
  Set Attribute : SetAttribute  AttributeName=IME_X|IME_Y|IME_Z  AttributeFrom=Dialog|Dialog|Dialog  AttributeValue=ME_X|ME_Y|ME_Z  AttributeTreatAsVector=1|1|1  EvaluatedAttributeValue={ ME_X;ME_Y;ME_Z}
  Input : PMIOPort  Port=1  Side=Left
  Output : PMIOPort  Port=2  Side=Right
  connections:
  Set Attribute/RConn1 -- Attribute Function/LConn1
  Output/RConn1 -- Attribute Function/RConn1
  Input/RConn1 -- Set Attribute/LConn1

== system NoC_4x4x3/LayerDown/Sitch3DXYZ10/RouteXYZ ==
  Attribute Function : Subsystem  LoadFcn=des.afb.attributefunction_support(gcb,'LoadFcn');  StartFcn=des.afb.attributefunction_support(gcb,'StartFcn');  mask(Attribute Function){OutputNamePrefix=out_}
      mask prompts: OutputNamePrefix "Prefix name"
      settings: CopyFcn=des.afb.attributefunction_support(gcb,'CopyFcn');  OpenFcn=des.afb.attributefunction_support(gcb,'OpenFcn');  ErrorFcn=des.afb.error_redirect
      mask Help: slhelp(gcbh)
      mask Display: image(des_iconLoad('attribFunction.jpg'),'center');
  Set Attribute : SetAttribute  AttributeName=IME_X|IME_Y|IME_Z  AttributeFrom=Dialog|Dialog|Dialog  AttributeValue=ME_X|ME_Y|ME_Z  AttributeTreatAsVector=1|1|1  EvaluatedAttributeValue={ ME_X;ME_Y;ME_Z}
  Input : PMIOPort  Port=1  Side=Left
  Output : PMIOPort  Port=2  Side=Right
  connections:
  Input/RConn1 -- Set Attribute/LConn1
  Output/RConn1 -- Attribute Function/RConn1
  Set Attribute/RConn1 -- Attribute Function/LConn1

== system NoC_4x4x3/LayerDown/Sitch3DXYZ11/RouteXYZ ==
  Attribute Function : Subsystem  LoadFcn=des.afb.attributefunction_support(gcb,'LoadFcn');  StartFcn=des.afb.attributefunction_support(gcb,'StartFcn');  mask(Attribute Function){OutputNamePrefix=out_}
      mask prompts: OutputNamePrefix "Prefix name"
      settings: CopyFcn=des.afb.attributefunction_support(gcb,'CopyFcn');  OpenFcn=des.afb.attributefunction_support(gcb,'OpenFcn');  ErrorFcn=des.afb.error_redirect
      mask Help: slhelp(gcbh)
      mask Display: image(des_iconLoad('attribFunction.jpg'),'center');
  Set Attribute : SetAttribute  AttributeName=IME_X|IME_Y|IME_Z  AttributeFrom=Dialog|Dialog|Dialog  AttributeValue=ME_X|ME_Y|ME_Z  AttributeTreatAsVector=1|1|1  EvaluatedAttributeValue={ ME_X;ME_Y;ME_Z}
  Input : PMIOPort  Port=1  Side=Left
  Output : PMIOPort  Port=2  Side=Right
  connections:
  Set Attribute/RConn1 -- Attribute Function/LConn1
  Output/RConn1 -- Attribute Function/RConn1
  Input/RConn1 -- Set Attribute/LConn1

== system NoC_4x4x3/LayerDown/Sitch3DXYZ12/RouteXYZ ==
  Attribute Function : Subsystem  LoadFcn=des.afb.attributefunction_support(gcb,'LoadFcn');  StartFcn=des.afb.attributefunction_support(gcb,'StartFcn');  mask(Attribute Function){OutputNamePrefix=out_}
      mask prompts: OutputNamePrefix "Prefix name"
      settings: CopyFcn=des.afb.attributefunction_support(gcb,'CopyFcn');  OpenFcn=des.afb.attributefunction_support(gcb,'OpenFcn');  ErrorFcn=des.afb.error_redirect
      mask Help: slhelp(gcbh)
      mask Display: image(des_iconLoad('attribFunction.jpg'),'center');
  Set Attribute : SetAttribute  AttributeName=IME_X|IME_Y|IME_Z  AttributeFrom=Dialog|Dialog|Dialog  AttributeValue=ME_X|ME_Y|ME_Z  AttributeTreatAsVector=1|1|1  EvaluatedAttributeValue={ ME_X;ME_Y;ME_Z}
  Input : PMIOPort  Port=1  Side=Left
  Output : PMIOPort  Port=2  Side=Right
  connections:
  Set Attribute/RConn1 -- Attribute Function/LConn1
  Output/RConn1 -- Attribute Function/RConn1
  Input/RConn1 -- Set Attribute/LConn1

== system NoC_4x4x3/LayerDown/Sitch3DXYZ13/RouteXYZ ==
  Attribute Function : Subsystem  LoadFcn=des.afb.attributefunction_support(gcb,'LoadFcn');  StartFcn=des.afb.attributefunction_support(gcb,'StartFcn');  mask(Attribute Function){OutputNamePrefix=out_}
      mask prompts: OutputNamePrefix "Prefix name"
      settings: CopyFcn=des.afb.attributefunction_support(gcb,'CopyFcn');  OpenFcn=des.afb.attributefunction_support(gcb,'OpenFcn');  ErrorFcn=des.afb.error_redirect
      mask Help: slhelp(gcbh)
      mask Display: image(des_iconLoad('attribFunction.jpg'),'center');
  Set Attribute : SetAttribute  AttributeName=IME_X|IME_Y|IME_Z  AttributeFrom=Dialog|Dialog|Dialog  AttributeValue=ME_X|ME_Y|ME_Z  AttributeTreatAsVector=1|1|1  EvaluatedAttributeValue={ ME_X;ME_Y;ME_Z}
  Input : PMIOPort  Port=1  Side=Left
  Output : PMIOPort  Port=2  Side=Right
  connections:
  Input/RConn1 -- Set Attribute/LConn1
  Output/RConn1 -- Attribute Function/RConn1
  Set Attribute/RConn1 -- Attribute Function/LConn1

== system NoC_4x4x3/LayerDown/Sitch3DXYZ14/RouteXYZ ==
  Attribute Function : Subsystem  LoadFcn=des.afb.attributefunction_support(gcb,'LoadFcn');  StartFcn=des.afb.attributefunction_support(gcb,'StartFcn');  mask(Attribute Function){OutputNamePrefix=out_}
      mask prompts: OutputNamePrefix "Prefix name"
      settings: CopyFcn=des.afb.attributefunction_support(gcb,'CopyFcn');  OpenFcn=des.afb.attributefunction_support(gcb,'OpenFcn');  ErrorFcn=des.afb.error_redirect
      mask Help: slhelp(gcbh)
      mask Display: image(des_iconLoad('attribFunction.jpg'),'center');
  Set Attribute : SetAttribute  AttributeName=IME_X|IME_Y|IME_Z  AttributeFrom=Dialog|Dialog|Dialog  AttributeValue=ME_X|ME_Y|ME_Z  AttributeTreatAsVector=1|1|1  EvaluatedAttributeValue={ ME_X;ME_Y;ME_Z}
  Input : PMIOPort  Port=1  Side=Left
  Output : PMIOPort  Port=2  Side=Right
  connections:
  Set Attribute/RConn1 -- Attribute Function/LConn1
  Output/RConn1 -- Attribute Function/RConn1
  Input/RConn1 -- Set Attribute/LConn1

== system NoC_4x4x3/LayerDown/Sitch3DXYZ15/RouteXYZ ==
  Attribute Function : Subsystem  LoadFcn=des.afb.attributefunction_support(gcb,'LoadFcn');  StartFcn=des.afb.attributefunction_support(gcb,'StartFcn');  mask(Attribute Function){OutputNamePrefix=out_}
      mask prompts: OutputNamePrefix "Prefix name"
      settings: CopyFcn=des.afb.attributefunction_support(gcb,'CopyFcn');  OpenFcn=des.afb.attributefunction_support(gcb,'OpenFcn');  ErrorFcn=des.afb.error_redirect
      mask Help: slhelp(gcbh)
      mask Display: image(des_iconLoad('attribFunction.jpg'),'center');
  Set Attribute : SetAttribute  AttributeName=IME_X|IME_Y|IME_Z  AttributeFrom=Dialog|Dialog|Dialog  AttributeValue=ME_X|ME_Y|ME_Z  AttributeTreatAsVector=1|1|1  EvaluatedAttributeValue={ ME_X;ME_Y;ME_Z}
  Input : PMIOPort  Port=1  Side=Left
  Output : PMIOPort  Port=2  Side=Right
  connections:
  Input/RConn1 -- Set Attribute/LConn1
  Output/RConn1 -- Attribute Function/RConn1
  Set Attribute/RConn1 -- Attribute Function/LConn1

== system NoC_4x4x3/LayerDown/Sitch3DXYZ2/RouteXYZ ==
  Attribute Function : Subsystem  LoadFcn=des.afb.attributefunction_support(gcb,'LoadFcn');  StartFcn=des.afb.attributefunction_support(gcb,'StartFcn');  mask(Attribute Function){OutputNamePrefix=out_}
      mask prompts: OutputNamePrefix "Prefix name"
      settings: CopyFcn=des.afb.attributefunction_support(gcb,'CopyFcn');  OpenFcn=des.afb.attributefunction_support(gcb,'OpenFcn');  ErrorFcn=des.afb.error_redirect
      mask Help: slhelp(gcbh)
      mask Display: image(des_iconLoad('attribFunction.jpg'),'center');
  Set Attribute : SetAttribute  AttributeName=IME_X|IME_Y|IME_Z  AttributeFrom=Dialog|Dialog|Dialog  AttributeValue=ME_X|ME_Y|ME_Z  AttributeTreatAsVector=1|1|1  EvaluatedAttributeValue={ ME_X;ME_Y;ME_Z}
  Input : PMIOPort  Port=1  Side=Left
  Output : PMIOPort  Port=2  Side=Right
  connections:
  Input/RConn1 -- Set Attribute/LConn1
  Output/RConn1 -- Attribute Function/RConn1
  Set Attribute/RConn1 -- Attribute Function/LConn1

== system NoC_4x4x3/LayerDown/Sitch3DXYZ3/RouteXYZ ==
  Attribute Function : Subsystem  LoadFcn=des.afb.attributefunction_support(gcb,'LoadFcn');  StartFcn=des.afb.attributefunction_support(gcb,'StartFcn');  mask(Attribute Function){OutputNamePrefix=out_}
      mask prompts: OutputNamePrefix "Prefix name"
      settings: CopyFcn=des.afb.attributefunction_support(gcb,'CopyFcn');  OpenFcn=des.afb.attributefunction_support(gcb,'OpenFcn');  ErrorFcn=des.afb.error_redirect
      mask Help: slhelp(gcbh)
      mask Display: image(des_iconLoad('attribFunction.jpg'),'center');
  Set Attribute : SetAttribute  AttributeName=IME_X|IME_Y|IME_Z  AttributeFrom=Dialog|Dialog|Dialog  AttributeValue=ME_X|ME_Y|ME_Z  AttributeTreatAsVector=1|1|1  EvaluatedAttributeValue={ ME_X;ME_Y;ME_Z}
  Input : PMIOPort  Port=1  Side=Left
  Output : PMIOPort  Port=2  Side=Right
  connections:
  Set Attribute/RConn1 -- Attribute Function/LConn1
  Output/RConn1 -- Attribute Function/RConn1
  Input/RConn1 -- Set Attribute/LConn1

== system NoC_4x4x3/LayerDown/Sitch3DXYZ4/RouteXYZ ==
  Attribute Function : Subsystem  LoadFcn=des.afb.attributefunction_support(gcb,'LoadFcn');  StartFcn=des.afb.attributefunction_support(gcb,'StartFcn');  mask(Attribute Function){OutputNamePrefix=out_}
      mask prompts: OutputNamePrefix "Prefix name"
      settings: CopyFcn=des.afb.attributefunction_support(gcb,'CopyFcn');  OpenFcn=des.afb.attributefunction_support(gcb,'OpenFcn');  ErrorFcn=des.afb.error_redirect
      mask Help: slhelp(gcbh)
      mask Display: image(des_iconLoad('attribFunction.jpg'),'center');
  Set Attribute : SetAttribute  AttributeName=IME_X|IME_Y|IME_Z  AttributeFrom=Dialog|Dialog|Dialog  AttributeValue=ME_X|ME_Y|ME_Z  AttributeTreatAsVector=1|1|1  EvaluatedAttributeValue={ ME_X;ME_Y;ME_Z}
  Input : PMIOPort  Port=1  Side=Left
  Output : PMIOPort  Port=2  Side=Right
  connections:
  Set Attribute/RConn1 -- Attribute Function/LConn1
  Output/RConn1 -- Attribute Function/RConn1
  Input/RConn1 -- Set Attribute/LConn1

== system NoC_4x4x3/LayerDown/Sitch3DXYZ5/RouteXYZ ==
  Attribute Function : Subsystem  LoadFcn=des.afb.attributefunction_support(gcb,'LoadFcn');  StartFcn=des.afb.attributefunction_support(gcb,'StartFcn');  mask(Attribute Function){OutputNamePrefix=out_}
      mask prompts: OutputNamePrefix "Prefix name"
      settings: CopyFcn=des.afb.attributefunction_support(gcb,'CopyFcn');  OpenFcn=des.afb.attributefunction_support(gcb,'OpenFcn');  ErrorFcn=des.afb.error_redirect
      mask Help: slhelp(gcbh)
      mask Display: image(des_iconLoad('attribFunction.jpg'),'center');
  Set Attribute : SetAttribute  AttributeName=IME_X|IME_Y|IME_Z  AttributeFrom=Dialog|Dialog|Dialog  AttributeValue=ME_X|ME_Y|ME_Z  AttributeTreatAsVector=1|1|1  EvaluatedAttributeValue={ ME_X;ME_Y;ME_Z}
  Input : PMIOPort  Port=1  Side=Left
  Output : PMIOPort  Port=2  Side=Right
  connections:
  Input/RConn1 -- Set Attribute/LConn1
  Output/RConn1 -- Attribute Function/RConn1
  Set Attribute/RConn1 -- Attribute Function/LConn1

== system NoC_4x4x3/LayerDown/Sitch3DXYZ6/RouteXYZ ==
  Attribute Function : Subsystem  LoadFcn=des.afb.attributefunction_support(gcb,'LoadFcn');  StartFcn=des.afb.attributefunction_support(gcb,'StartFcn');  mask(Attribute Function){OutputNamePrefix=out_}
      mask prompts: OutputNamePrefix "Prefix name"
      settings: CopyFcn=des.afb.attributefunction_support(gcb,'CopyFcn');  OpenFcn=des.afb.attributefunction_support(gcb,'OpenFcn');  ErrorFcn=des.afb.error_redirect
      mask Help: slhelp(gcbh)
      mask Display: image(des_iconLoad('attribFunction.jpg'),'center');
  Set Attribute : SetAttribute  AttributeName=IME_X|IME_Y|IME_Z  AttributeFrom=Dialog|Dialog|Dialog  AttributeValue=ME_X|ME_Y|ME_Z  AttributeTreatAsVector=1|1|1  EvaluatedAttributeValue={ ME_X;ME_Y;ME_Z}
  Input : PMIOPort  Port=1  Side=Left
  Output : PMIOPort  Port=2  Side=Right
  connections:
  Set Attribute/RConn1 -- Attribute Function/LConn1
  Output/RConn1 -- Attribute Function/RConn1
  Input/RConn1 -- Set Attribute/LConn1

== system NoC_4x4x3/LayerDown/Sitch3DXYZ7/RouteXYZ ==
  Attribute Function : Subsystem  LoadFcn=des.afb.attributefunction_support(gcb,'LoadFcn');  StartFcn=des.afb.attributefunction_support(gcb,'StartFcn');  mask(Attribute Function){OutputNamePrefix=out_}
      mask prompts: OutputNamePrefix "Prefix name"
      settings: CopyFcn=des.afb.attributefunction_support(gcb,'CopyFcn');  OpenFcn=des.afb.attributefunction_support(gcb,'OpenFcn');  ErrorFcn=des.afb.error_redirect
      mask Help: slhelp(gcbh)
      mask Display: image(des_iconLoad('attribFunction.jpg'),'center');
  Set Attribute : SetAttribute  AttributeName=IME_X|IME_Y|IME_Z  AttributeFrom=Dialog|Dialog|Dialog  AttributeValue=ME_X|ME_Y|ME_Z  AttributeTreatAsVector=1|1|1  EvaluatedAttributeValue={ ME_X;ME_Y;ME_Z}
  Input : PMIOPort  Port=1  Side=Left
  Output : PMIOPort  Port=2  Side=Right
  connections:
  Input/RConn1 -- Set Attribute/LConn1
  Output/RConn1 -- Attribute Function/RConn1
  Set Attribute/RConn1 -- Attribute Function/LConn1
